simulink model "MPCRoadTracking"  (Simulink 9.0)
settings: Solver=VariableStepAuto  StartTime=0.0  StopTime=300  RelTol=1e-3
libraries: Solver_SF x1
settings Model: Creator=auto  LastModifiedBy=auto
settings DataIOCC: SaveFormat=Dataset
settings OptimizationCC: LifeSpan=auto
settings DebuggingCC: UnderspecifiedInitializationDetection=Simplified  MergeDetectMultiDrivingBlocksExec=error  SFUnexpectedBacktrackingDiag=error  SFNoUnconditionalDefaultTransitionDiag=error  SFExecutionAtInitializationDiag=warning
settings HardwareCC: ProdBitPerPointer=64  ProdBitPerSizeT=64  ProdBitPerPtrDiffT=64  ProdLargestAtomicFloat=Float  ProdIntDivRoundTo=Zero  ProdEndianess=LittleEndian  ProdWordSize=64  ProdHWDeviceType=Intel->x86-64 (Windows64)
settings ModelReferenceCC: PropagateSignalLabelsOutOfModel=on
settings CodeAppCC: StateflowObjectComments=off
settings GRTTargetCC: TargetLangStandard=C99 (ISO)
settings ConfigComp: CovMetricSettings=dwe  CovHtmlReporting=off  CovSaveCumulativeToWorkspaceVar=off  CovSaveSingleToWorkspaceVar=off  CovExternalEMLEnable=on

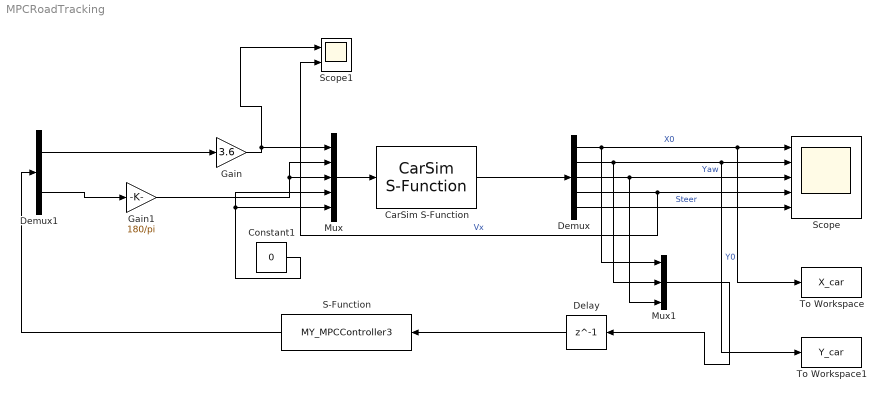
== system MPCRoadTracking ==
  CarSim S-Function : Solver_SF/CarSim S-Function  Priority=1  VehicleCode=i_i  SIMFILE=simfile.sim
  Constant1 : Constant  Value=0
  Delay : Delay  DelayLength=1  InitialCondition=0
  Demux : Demux  Outputs=5
  Demux1 : Demux  Outputs=2
  Gain : Gain  Gain=3.6
  Gain1 : Gain  Gain=180/pi
  Mux : Mux  Inputs=5
  Mux1 : Mux  Inputs=3
  S-Function : S-Function  FunctionName=MY_MPCController3  SFunctionDeploymentMode=off  EnableBusSupport=off
  Scope : Scope  NumInputPorts=5
  Scope1 : Scope  NumInputPorts=2
  To Workspace : ToWorkspace  VariableName=X_car  SaveFormat=Timeseries  SampleTime=-1
  To Workspace1 : ToWorkspace  VariableName=Y_car  SaveFormat=Timeseries  SampleTime=-1
  wires:
  Mux/1 -> CarSim S-Function/1
  CarSim S-Function/1 -> Demux/1
  Demux/1 -> Mux1/1, To Workspace/1, Scope/1  "X0"
  Demux/2 -> Mux1/2, To Workspace1/1, Scope/2  "Y0"
  Demux/3 -> Mux1/3, Scope/3  "Yaw"
  Demux/4 -> Scope1/2, Scope/4  "Vx"
  Demux/5 -> Scope/5  "Steer"
  Mux1/1 -> Delay/1
  Constant1/1 -> Mux/4, Mux/5
  Gain/1 -> Scope1/1, Mux/1
  Delay/1 -> S-Function/1
  S-Function/1 -> Demux1/1
  Demux1/1 -> Gain/1
  Demux1/2 -> Gain1/1
  Gain1/1 -> Mux/3, Mux/2
